simulink model "buck_open_loop"  (Simulink 9.0)
settings: Solver=ode45  StartTime=0.0  StopTime=0.01  MaxStep=0.1e-6  RelTol=1e-3  EnableMultiTasking=on
libraries: simulink x1
settings Model: Creator=kamyar  LastModifiedBy="ASUS  N551JW"
settings DataIOCC: LimitDataPoints=on  SignalLoggingSaveFormat=ModelDataLogs
settings DebuggingCC: SaveWithParameterizedLinksMsg=none  SignalResolutionControl=TryResolveAllWithWarning  MultiTaskDSMMsg=warning  MultiTaskCondExecSysMsg=none  AllowSymbolicDim=off  StrictBusMsg=None
settings HardwareCC: ProdBitPerPointer=64  ProdBitPerSizeT=64  ProdBitPerPtrDiffT=64  ProdLargestAtomicFloat=Float  ProdIntDivRoundTo=Zero  ProdEndianess=LittleEndian  ProdWordSize=64  ProdHWDeviceType=Intel->x86-64 (Windows64)  TargetUnknown=on
settings GRTTargetCC: CombineOutputUpdateFcns=off  GRTInterface=on

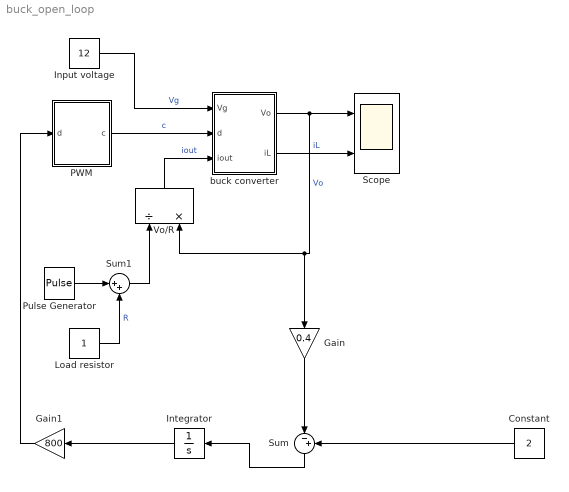
== system buck_open_loop ==
  Constant : Constant  Value=2
  Gain : Gain  Gain=0.4
  Gain1 : Gain  Gain=800
  Input voltage : Constant  Value=12
  Integrator : Integrator
  Load resistor : Constant
  PWM : Subsystem
  Pulse Generator : DiscretePulseGenerator  PulseType=Time based  Period=0.002  PulseWidth=50
  Scope : Scope  NumInputPorts=2
  Sum : Sum  Inputs=|-+
  Sum1 : Sum  Inputs=|++
  Vo/R : Product  Inputs=/*  SaturateOnIntegerOverflow=on  RndMeth=Zero  InputSameDT=on  OutDataTypeStr=Inherit: Same as first input
  buck converter : Subsystem
  wires:
  Input voltage/1 -> buck converter/1(Vg)  "Vg"
  buck converter/1(Vo) -> Gain/1, Vo/R/2, Scope/1  "Vo"
  buck converter/2(iL) -> Scope/2  "iL"
  PWM/1(c) -> buck converter/2(d)  "c"
  Vo/R/1 -> buck converter/3(iout)  "iout"
  Constant/1 -> Sum/2
  Gain/1 -> Sum/1
  Sum/1 -> Integrator/1
  Integrator/1 -> Gain1/1
  Gain1/1 -> PWM/1(d)
  Sum1/1 -> Vo/R/1
  Load resistor/1 -> Sum1/2  "R"
  Pulse Generator/1 -> Sum1/1

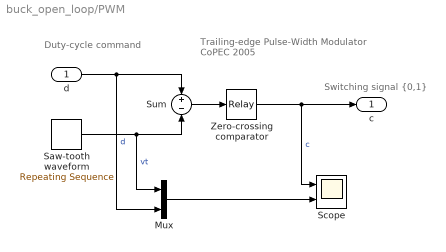
== system buck_open_loop/PWM ==
  note: Duty-cycle
      | command
  note: Switching signal {0,1}
  note: Trailing-edge Pulse-Width Modulator
      | CoPEC 2005
  d : Inport
  Mux : Mux  Inputs=2
  Saw-tooth waveform : simulink/Sources/Repeating Sequence  rep_seq_t=[0 0.001e-5 1e-5]  rep_seq_y=[1 0 1]
  Scope : Scope  NumInputPorts=2
  Sum : Sum  Inputs=+|-  SaturateOnIntegerOverflow=on  InputSameDT=on  OutDataTypeStr=Inherit: Same as first input
  Zero-crossing comparator : Relay
  c : Outport
  wires:
  Saw-tooth waveform/1 -> Mux/1, Sum/2  "vt"
  d/1 -> Mux/2, Sum/1  "d"
  Zero-crossing comparator/1 -> c/1, Scope/1  "c"
  Sum/1 -> Zero-crossing comparator/1
  Mux/1 -> Scope/2

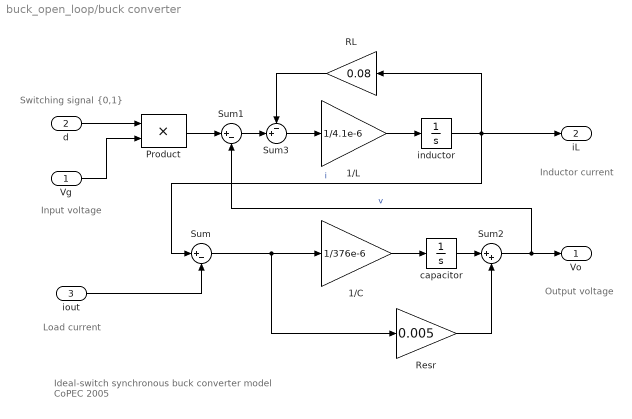
== system buck_open_loop/buck converter ==
  note: Load current
  note: Input voltage
  note: Inductor current
  note: Output voltage
  note: Switching signal {0,1}
  note: Ideal-switch synchronous buck converter model
      | CoPEC 2005
  Vg : Inport
  d : Inport  Port=2
  iout : Inport  Port=3
  1/C : Gain  Gain=1/376e-6  SaturateOnIntegerOverflow=on  OutDataTypeStr=Inherit: Same as input  ParamDataTypeStr=Inherit: Same as input
  1/L : Gain  Gain=1/4.1e-6  SaturateOnIntegerOverflow=on  OutDataTypeStr=Inherit: Same as input  ParamDataTypeStr=Inherit: Same as input
  Product : Product  SaturateOnIntegerOverflow=on  RndMeth=Zero  InputSameDT=on  OutDataTypeStr=Inherit: Same as first input
  RL : Gain  Gain=0.08  SaturateOnIntegerOverflow=on  OutDataTypeStr=Inherit: Same as input  ParamDataTypeStr=Inherit: Same as input
  Resr : Gain  Gain=0.005  SaturateOnIntegerOverflow=on  OutDataTypeStr=Inherit: Same as input  ParamDataTypeStr=Inherit: Same as input
  Sum : Sum  Inputs=|+-  SaturateOnIntegerOverflow=on  InputSameDT=on  OutDataTypeStr=Inherit: Same as first input
  Sum1 : Sum  Inputs=|+-  SaturateOnIntegerOverflow=on  InputSameDT=on  OutDataTypeStr=Inherit: Same as first input
  Sum2 : Sum  Inputs=|++  SaturateOnIntegerOverflow=on  InputSameDT=on  OutDataTypeStr=Inherit: Same as first input
  Sum3 : Sum  Inputs=-+|  SaturateOnIntegerOverflow=on  InputSameDT=on  OutDataTypeStr=Inherit: Same as first input
  capacitor : Integrator
  inductor : Integrator
  Vo : Outport
  iL : Outport  Port=2
  wires:
  iout/1 -> Sum/2
  d/1 -> Product/1
  Resr/1 -> Sum2/2
  capacitor/1 -> Sum2/1
  Sum3/1 -> 1/L/1
  RL/1 -> Sum3/1
  Sum1/1 -> Sum3/2
  Sum2/1 -> Sum1/2, Vo/1  "v"
  Product/1 -> Sum1/1
  inductor/1 -> Sum/1, RL/1, iL/1  "i"
  1/L/1 -> inductor/1
  Sum/1 -> 1/C/1, Resr/1
  1/C/1 -> capacitor/1
  Vg/1 -> Product/2
